simulink model "DKHD_CH29a_3_1_S"  (Simulink 8.5)
settings: Solver=ode45  StartTime=0.0  StopTime=100  RelTol=1e-3
libraries: fuzblock x1
settings Model: Creator=home  LastModifiedBy=Admin  CovSFcnEnable=off
settings SolverCC: ZeroCrossControl=DisableAll  ZeroCrossAlgorithm=Adaptive
settings DataIOCC: SignalLoggingSaveFormat=Dataset
settings DebuggingCC: MultiTaskDSMMsg=warning  MultiTaskCondExecSysMsg=none  FcnCallInpInsideContextMsg=EnableAllAsWarning
settings GRTTargetCC: CombineOutputUpdateFcns=on  GRTInterface=off

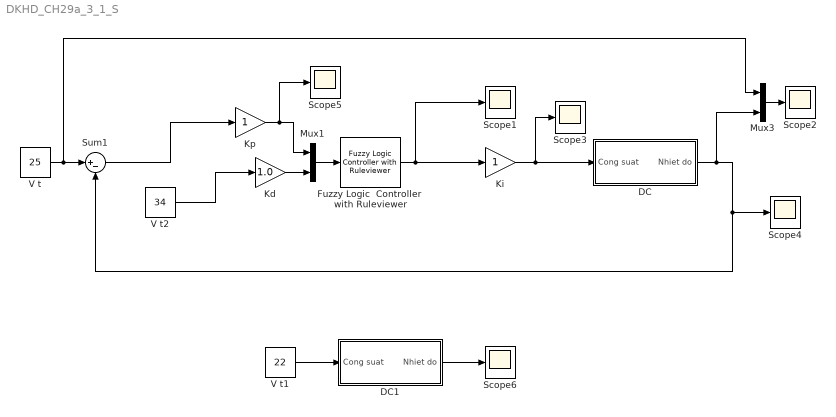
== system DKHD_CH29a_3_1_S ==
  DC : Subsystem
  DC1 : Subsystem
  Fuzzy Logic  Controller  with Ruleviewer : fuzblock/Fuzzy Logic  Controller  with Ruleviewer  fismatrix=DKHD_CH29a_3_1_F  Ts=2
  Kd : Gain  Gain=1.0
  Ki : Gain
  Kp : Gain
  Mux1 : Mux  Inputs=2
  Mux3 : Mux  Inputs=2
  Scope{1..6} (6 alike) : Scope
      Scope2 settings: TimeRange=100  YMin=0  YMax=35
      Scope3 settings: SaveName=ScopeData2
      Scope4 settings: SaveName=ScopeData3
      Scope5 settings: SaveName=ScopeData4
      Scope6 settings: SaveName=ScopeData5
  Sum1 : Sum  Inputs=|+-
  V t : Constant  Value=25
  V t1 : Constant  Value=22
  V t2 : Constant  Value=34
  wires:
  V t/1 -> Sum1/1, Mux3/1
  DC/1(Nhiet do) -> Mux3/2, Scope4/1, Sum1/2
  Fuzzy Logic  Controller  with Ruleviewer/1 -> Scope1/1, Ki/1
  Mux1/1 -> Fuzzy Logic  Controller  with Ruleviewer/1
  Ki/1 -> Scope3/1, DC/1(Cong suat)
  Kp/1 -> Scope5/1, Mux1/1
  Kd/1 -> Mux1/2
  Mux3/1 -> Scope2/1
  V t1/1 -> DC1/1(Cong suat)
  DC1/1(Nhiet do) -> Scope6/1
  Sum1/1 -> Kp/1
  V t2/1 -> Kd/1

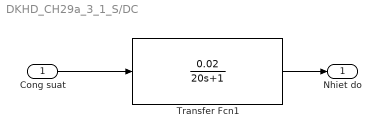
== system DKHD_CH29a_3_1_S/DC ==
  Cong suat : Inport
  Transfer Fcn1 : TransferFcn  Numerator=[0.02]  Denominator="[20  1]"
  Nhiet do : Outport
  wires:
  Cong suat/1 -> Transfer Fcn1/1
  Transfer Fcn1/1 -> Nhiet do/1

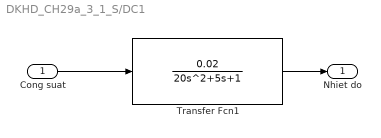
== system DKHD_CH29a_3_1_S/DC1 ==
  Cong suat : Inport
  Transfer Fcn1 : TransferFcn  Numerator=[0.02]  Denominator="[20  5  1]"
  Nhiet do : Outport
  wires:
  Cong suat/1 -> Transfer Fcn1/1
  Transfer Fcn1/1 -> Nhiet do/1
